simulink model "second_order_system"  (R2016a)
settings: Solver=VariableStepAuto  StartTime=0.0  StopTime=30  MaxStep=1e-2  RelTol=1e-3
values from neighbouring files (symbols this model uses):
  K = 1    [second_order_system.m]    (also in second_order_system_init.m; test_exp.m)
  wn = 1    [second_order_system.m]    (also in second_order_system_init.m)
  z = linspace(0,1,100)'    [overshoot.m]    (also in overshoot_to_damping.m = sqrt(log(PO/100)^2/(pi^2+log(PO/100)^2)); second_order_system.m = 0.5; second_order_system_init.m = 0.5)
settings Model: Creator=alexalcocer  LastModifiedBy=alexalcocer

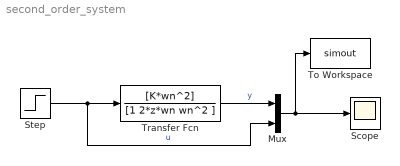
== system second_order_system ==
  Mux : Mux  Inputs=2
  Scope : Scope
  Step : Step  SampleTime=0
  To Workspace : ToWorkspace  VariableName=simout  SaveFormat=Timeseries  SampleTime=-1
  Transfer Fcn : TransferFcn  Numerator=[K*wn^2]  Denominator=[1 2*z*wn wn^2 ]
  wires:
  Mux/1 -> To Workspace/1, Scope/1
  Transfer Fcn/1 -> Mux/1  "y"
  Step/1 -> Transfer Fcn/1, Mux/2  "u"
